simulink model "Mechatronics"  (R2020b)
settings: Solver=VariableStepAuto  StartTime=0.0  StopTime=5  RelTol=1e-3
libraries: pid_lib x1
settings Model: Creator=Simon Gebraad  LastModifiedBy=Simon Gebraad

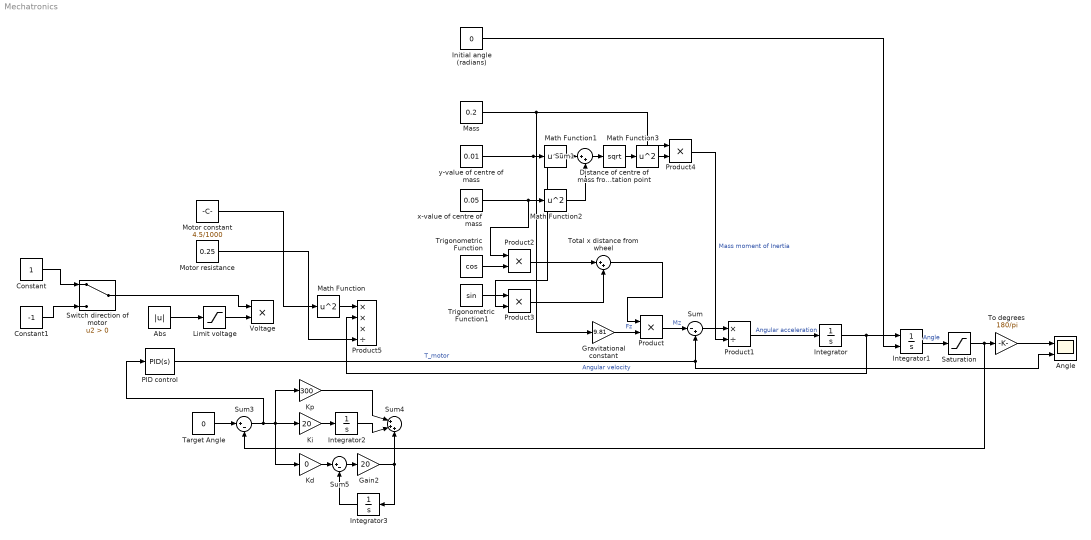
== system Mechatronics ==
  Abs : Abs
  Angle : Scope  NumInputPorts=2
  Constant : Constant
  Constant1 : Constant  Value=-1
  "Distance of centre of mass from rotation point " : Sqrt  SaturateOnIntegerOverflow=on
  Gain2 : Gain  Gain=20
  Gravitational constant : Gain  Gain=9.81
  Initial angle (radians) : Constant  Value=0
  Integrator : Integrator
  Integrator1 : Integrator  InitialConditionSource=external
  Integrator2 : Integrator
  Integrator3 : Integrator
  Kd : Gain  Gain=0
  Ki : Gain  Gain=20
  Kp : Gain  Gain=300
  Limit voltage : Saturate  UpperLimit=16  LowerLimit=4
  Mass : Constant  Value=0.2
  Math Function{,1..3} (4 alike) : Math  Operator=square  SaturateOnIntegerOverflow=on
  Motor constant : Constant  Value=4.5/1000
  Motor resistance : Constant  Value=0.25
  PID control : pid_lib/PID Controller  Controller=PID  Form=Parallel  TimeDomain=Continuous-time  UseExternalTs=off  SampleTime=-1  IntegratorMethod=Forward Euler  FilterMethod=Forward Euler  ControllerParametersSource=internal  P=3.60881190211891  I=34.4753313656519  D=0.0933922260980466  UseFilter=on  N=20796.0504924641  TunerSelectOption=Transfer Function Based (PID Tuner App)  InitialConditionSource=internal  InitialConditionForIntegrator=0  InitialConditionForFilter=0  DifferentiatorICPrevScaledInput=0  ExternalReset=none  TrackingMode=off  Kt=1  LimitOutput=off  SatLimitsSource=internal  UpperSaturationLimit=inf  LowerSaturationLimit=-inf  LinearizeAsGain=on  AntiWindupMode=none  Kb=1  POutMin=[]  POutMax=[]  IOutMin=[]  IOutMax=[]  DOutMin=[]  DOutMax=[]  NOutMin=[]  NOutMax=[]  SumOutMin=[]  SumOutMax=[]  SaturationOutMin=[]  SaturationOutMax=[]  PParamMin=[]  PParamMax=[]  IParamMin=[]  IParamMax=[]  DParamMin=[]  DParamMax=[]  NParamMin=[]  NParamMax=[]  KbParamMin=[]  KbParamMax=[]  KtParamMin=[]  KtParamMax=[]  KbOutMin=[]  KbOutMax=[]  KtOutMin=[]  KtOutMax=[]  IntegratorOutMin=[]  IntegratorOutMax=[]  FilterOutMin=[]  FilterOutMax=[]  SumI1OutMin=[]  SumI1OutMax=[]  SumI2OutMin=[]  SumI2OutMax=[]  SumI3OutMin=[]  SumI3OutMax=[]  SumI4OutMin=[]  SumI4OutMax=[]  SumDOutMin=[]  SumDOutMax=[]  DifferentiatorOutMin=[]  DifferentiatorOutMax=[]  FilterDiffOutCoefMin=[]  FilterDiffOutCoefMax=[]  ReciprocalOutMin=[]  ReciprocalOutMax=[]  SumDenOutMin=[]  SumDenOutMax=[]  SumNumOutMin=[]  SumNumOutMax=[]  DivideOutMin=[]  DivideOutMax=[]  UdiffTsProdOutMin=[]  UdiffTsProdOutMax=[]  NTsProdOutMin=[]  NTsProdOutMax=[]  UintegralTsProdOutMin=[]  UintegralTsProdOutMax=[]  UngainTsProdOutMin=[]  UngainTsProdOutMax=[]  IntegratorContinuousStateAttributes=''  IntegratorStateMustResolveToSignalObject=off  IntegratorRTWStateStorageClass=Auto  FilterContinuousStateAttributes=''  FilterStateMustResolveToSignalObject=off  FilterRTWStateStorageClass=Auto  ParallelPVariant=InternalParameters  IdealPVariant=Disabled  IVariant=InternalParameters  DVariant=InternalParameters  IntegratorVariant=Continuous  SatVariant=Disabled  AWVariant=Passthrough  PCopyVariant=Disabled  TRVariant=Disabled  FdbkBlocksVariant=Forward  IdealPFdbkVariant=Disabled  SatFdbkVariant=Disabled  DerivativeFilterVariant=ContFilter  NVariant=InternalParameters  NCopyVariant=Disabled  FilterICVariant=InternalICsFilter  IntegratorICVariant=InternalICs  ExternalResetVariant=Disabled  TRSumVariant=Passthrough  SumFdbkVariant=Disabled  SumVariant=Sum_PID  TsampFilterVariant=InternalTs  TsampNgainVariant=Passthrough  TsampIntegralVariant=Passthrough  ExternalSaturationOutDataTypeStr=Inherit: Same as second input
  Product{,2..4} (4 alike) : Product
  Product1 : Product  Inputs=*/
  Product5 : Product  Inputs=***/
  Saturation : Saturate  UpperLimit=pi  LowerLimit=-pi
  Sum : Sum  Inputs=|-+
  Sum1 : Sum  Inputs=|++
  Sum3 : Sum  Inputs=|+-
  Sum4 : Sum  Inputs=|+++
  Sum5 : Sum  Inputs=|+-
  Switch direction of motor : Switch  Criteria=u2 > Threshold
  Target Angle : Constant  Value=0
  To degrees : Gain  Gain=180/pi
  Total x distance from wheel : Sum  Inputs=|++
  Trigonometric Function : Trigonometry  Operator=cos
  Trigonometric Function1 : Trigonometry
  Voltage : Product
  x-value of centre of mass : Constant  Value=0.05
  y-value of centre of mass : Constant  Value=0.01
  wires:
  Mass/1 -> Product4/1, Gravitational constant/1
  Gravitational constant/1 -> Product/2  "Fz"
  Product/1 -> Sum/1  "Mz"
  Sum/1 -> Product1/1
  Integrator/1 -> Product5/2, Integrator1/1  "Angular velocity"
  Integrator1/1 -> Saturation/1  "Angle"
  Target Angle/1 -> Sum3/1
  Sum3/1 -> PID control/1, Kp/1, Kd/1, Ki/1
  Ki/1 -> Integrator2/1
  Kp/1 -> Sum4/1
  Integrator2/1 -> Sum4/2
  Kd/1 -> Sum5/1
  Sum5/1 -> Gain2/1
  Gain2/1 -> Integrator3/1, Sum4/3
  Integrator3/1 -> Sum5/2
  Trigonometric Function/1 -> Product2/2
  x-value of centre of mass/1 -> Math Function2/1, Product2/1
  Trigonometric Function1/1 -> Product3/1
  Product2/1 -> Total x distance from wheel/1
  Product3/1 -> Total x distance from wheel/2
  Total x distance from wheel/1 -> Product/1
  Constant/1 -> Switch direction of motor/1
  Constant1/1 -> Switch direction of motor/3
  Switch direction of motor/1 -> Voltage/1
  Motor constant/1 -> Math Function/1
  Math Function/1 -> Product5/1
  Motor resistance/1 -> Product5/4
  y-value of centre of mass/1 -> Product3/2, Math Function1/1
  Math Function1/1 -> Sum1/1
  Math Function2/1 -> Sum1/2
  Sum1/1 -> "Distance of centre of mass from rotation point "/1
  "Distance of centre of mass from rotation point "/1 -> Math Function3/1
  Math Function3/1 -> Product4/2
  Product4/1 -> Product1/2  "Mass moment of Inertia"
  Abs/1 -> Limit voltage/1
  Initial angle (radians)/1 -> Integrator1/2
  To degrees/1 -> Angle/1
  Saturation/1 -> Sum3/2, To degrees/1
  Product1/1 -> Integrator/1  "Angular acceleration"
  PID control/1 -> Sum/2, Angle/2  "T_motor"
  Limit voltage/1 -> Voltage/2
